simulink model "auto_vehicle_moving_test_01"  (R2026a)
settings: Solver=FixedStepDiscrete
model workspace (MAT data in the model file):
  firstWarning = 1
  originalScenarioChecksum = '0B1B60020F3A3463CBBEA95029416C8C'
libraries: drivingscenarioandsensors x1
settings Model: Creator=pavanreddy  LastModifiedBy=pavanreddy

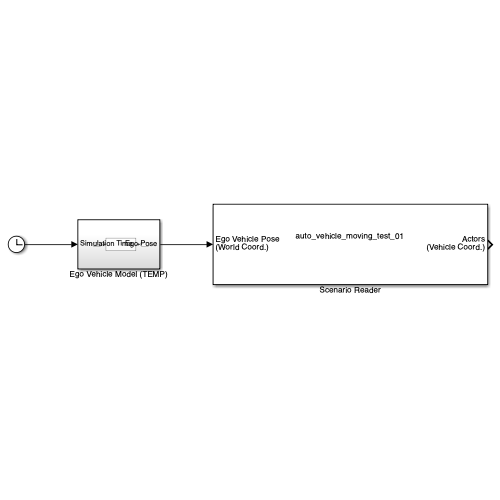
[thumbnail: Simulink's stored preview of the top-level diagram]
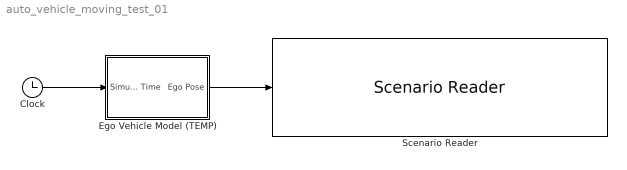
== system auto_vehicle_moving_test_01 ==
  Clock : Clock
  Ego Vehicle Model (TEMP) : Subsystem
  Scenario Reader : drivingscenarioandsensors/Scenario Reader  ScenarioSource=From file  ScenarioFileName=/Users/pavanreddy/Documents/MATLAB/LidarAnalysis/scenarios/auto_vehicle_moving_test_01.mat  ScenarioVariableName=scenario  OutputCoordinateSystem=Vehicle coordinates  EgoVehicleSource=Input port  EgoVehicleActorID=1  OrientVehiclesOnRoad=off  OutputEgoVehiclePose=off  OutputEgoVehicleState=off  SampleTime=0.1  LaneBoundaryOutput=None  LaneBoundaryDistance=0:0.5:9.5  LaneBoundaryLocation=Center of lane markings  BusNameSource=Auto  BusName=BusActors  BusNumActorsSource=Scenario  BusNumActors=100  BusName2Source=Auto  BusName2=BusLaneBoundaries  BusNumLaneBoundariesSource=Scenario  BusNumLaneBoundaries=10  BusName3Source=Auto  BusName3=BusEgoActor  BusName4Source=Auto  BusName4=BusEgoState  ShowCoordinateLabels=on  SimulateUsing=Interpreted execution
  wires:
  Clock/1 -> Ego Vehicle Model (TEMP)/1(Simulation Time)
  Ego Vehicle Model (TEMP)/1(Ego Pose) -> Scenario Reader/1

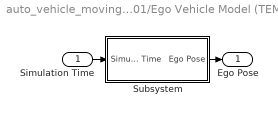
== system auto_vehicle_moving_test_01/Ego Vehicle Model (TEMP) ==
  Simulation Time : Inport
  Subsystem : Subsystem
  Ego Pose : Outport
  wires:
  Simulation Time/1 -> Subsystem/1(Simulation Time)
  Subsystem/1(Ego Pose) -> Ego Pose/1

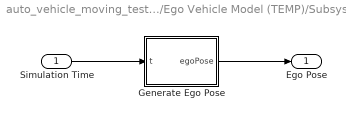
== system auto_vehicle_moving_test_01/Ego Vehicle Model (TEMP)/Subsystem ==
  Simulation Time : Inport
  Generate Ego Pose : MATLAB Function  TreatAsAtomicUnit=on
  Ego Pose : Outport
  wires:
  Simulation Time/1 -> Generate Ego Pose/1(t)
  Generate Ego Pose/1(egoPose) -> Ego Pose/1

== matlab function auto_vehicle_moving_test_01/Ego Vehicle Model (TEMP)/Subsystem/Generate Ego Pose ==
  data: t input double size=1; egoPose output Bus: EgoPoseBus
function egoPose = fcn(t)
%#codegen

% Initial ego vehicle state from Driving Scenario Designer
x0 = 31.7;
y0 = 31.6;
z0 = 0.0;

% Initial heading
yaw = -90.3504;

% Temporary test speed
speed = 10.0;   % m/s

% World-coordinate velocity
vx = speed * cosd(yaw);
vy = speed * sind(yaw);
vz = 0.0;

% Actor ID
egoPose.ActorID = 1;

% Position
egoPose.Position = [ ...
    x0 + vx*t; ...
    y0 + vy*t; ...
    z0];

% Velocity
egoPose.Velocity = [vx; vy; vz];
% Orientation
egoPose.Roll = 0.0;
egoPose.Pitch = 0.0;
egoPose.Yaw = yaw;

% Angular velocity
egoPose.AngularVelocity = [0.0; 0.0; 0.0];
